simulink model "Main_Model_Braking_Demo"  (R2023b)
settings: Solver=FixedStepDiscrete  StartTime=0.0  StopTime=10.0  RelTol=1e-3
settings Model: Creator=E8KUAVE  LastModifiedBy=E8KUAVE
settings OptimizationCC: DefaultParameterBehavior=Inlined  EnhancedBackFolding=on  PassReuseOutputArgsAs=Individual arguments  ZeroExternalMemoryAtStartup=off  ZeroInternalMemoryAtStartup=off  OptimizeBlockOrder=speed  DifferentSizesBufferReuse=on  OptimizationCustomize=off  EfficientTunableParamExpr=on
settings DebuggingCC: ParameterTunabilityLossMsg=error
settings HardwareCC: ProdBitPerPointer=32  ProdBitPerSizeT=32  ProdBitPerPtrDiffT=32  ProdLargestAtomicInteger=Long  ProdLargestAtomicFloat=Double  ProdWordSize=32  ProdHWDeviceType=ARM Compatible->ARM Cortex-M
settings SFSimCC: MATLABDynamicMemAlloc=off  SimTargetLang=C++
settings RTWCC: Description=Embedded Coder  SystemTargetFile=ert.tlc  GenCodeOnly=on  TemplateMakefile=ert_default_tmf  Toolchain=MinGW64 | gmake (64-bit Windows)  DataTypeReplacement=CDataTypesFixedWidth  TargetLang=C++
settings CodeAppCC: ForceParamTrailComments=on  IgnoreCustomStorageClasses=off  OperatorAnnotations=on  SimulinkDataObjDesc=on  SFDataObjDesc=on  InsertBlockDesc=on
settings ERTTargetCC: TargetLangStandard=C++11 (ISO)  GenerateSampleERTMain=on  CodeInterfacePackaging=C++ class  PurelyIntegerCode=on  SupportNonFinite=off  InlinedParameterPlacement=NonHierarchical  RootIOFormat=Structure reference  ERTCustomFileTemplate=example_file_process.tlc  MaxIdInt64=INT64_MAX  MinIdInt64=INT64_MIN  MaxIdUint64=UINT64_MAX  MaxIdInt32=INT32_MAX  MinIdInt32=INT32_MIN  MaxIdUint32=UINT32_MAX  MaxIdInt16=INT16_MAX  MinIdInt16=INT16_MIN  MaxIdUint16=UINT16_MAX  MaxIdInt8=INT8_MAX  MinIdInt8=INT8_MIN  MaxIdUint8=UINT8_MAX

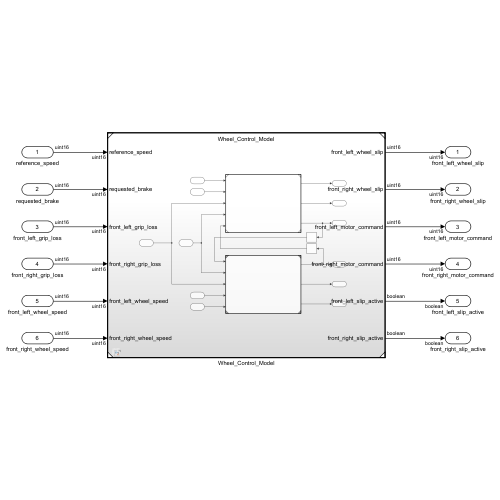
[thumbnail: Simulink's stored preview of the top-level diagram]
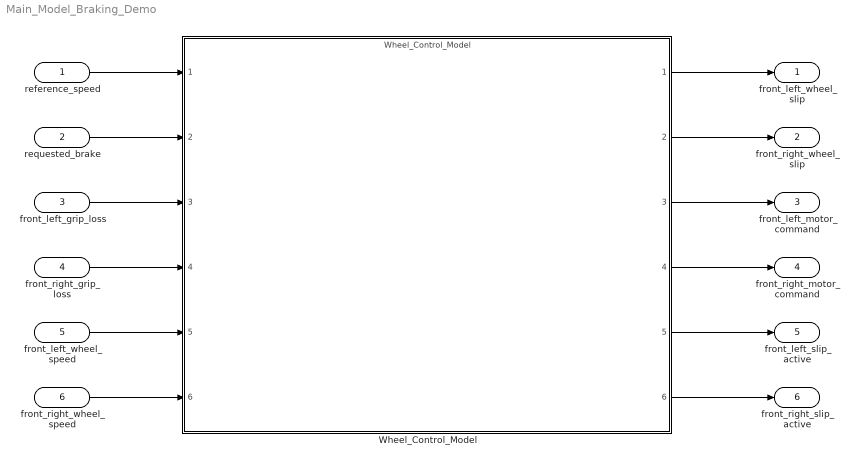
== system Main_Model_Braking_Demo ==
  reference_speed : Inport  OutDataTypeStr=uint16
  requested_brake : Inport  Port=2  OutDataTypeStr=uint16
  front_left_grip_loss : Inport  Port=3  OutDataTypeStr=uint16
  front_right_grip_loss : Inport  Port=4  OutDataTypeStr=uint16
  front_left_wheel_speed : Inport  Port=5  OutDataTypeStr=uint16
  front_right_wheel_speed : Inport  Port=6  OutDataTypeStr=uint16
  Wheel_Control_Model : ModelReference  ModelNameDialog=Wheel_Control_Model.slx  SimulationMode=Normal  ModelReferenceVersion=1.14
  front_left_wheel_slip : Outport  OutDataTypeStr=uint16
  front_right_wheel_slip : Outport  Port=2  OutDataTypeStr=uint16
  front_left_motor_command : Outport  Port=3  OutDataTypeStr=uint16
  front_right_motor_command : Outport  Port=4  OutDataTypeStr=uint16
  front_left_slip_active : Outport  Port=5  OutDataTypeStr=boolean
  front_right_slip_active : Outport  Port=6  OutDataTypeStr=boolean
  wires:
  reference_speed/1 -> Wheel_Control_Model/1
  requested_brake/1 -> Wheel_Control_Model/2
  front_left_grip_loss/1 -> Wheel_Control_Model/3
  front_right_grip_loss/1 -> Wheel_Control_Model/4
  front_left_wheel_speed/1 -> Wheel_Control_Model/5
  front_right_wheel_speed/1 -> Wheel_Control_Model/6
  Wheel_Control_Model/1 -> front_left_wheel_slip/1
  Wheel_Control_Model/2 -> front_right_wheel_slip/1
  Wheel_Control_Model/3 -> front_left_motor_command/1
  Wheel_Control_Model/4 -> front_right_motor_command/1
  Wheel_Control_Model/5 -> front_left_slip_active/1
  Wheel_Control_Model/6 -> front_right_slip_active/1
